simulink model "conversion"  (Simulink 10.1)
settings: Solver=FixedStepDiscrete  StartTime=0.0  StopTime=10.0  FixedStep=0.1  RelTol=1e-3  EnableMultiTasking=on
settings Model: Creator=Demos  LastModifiedBy=MaximeBe
settings DataIOCC: LimitDataPoints=on  SignalLoggingSaveFormat=ModelDataLogs
settings OptimizationCC: ExpressionDepthLimit=2147483647  ZeroExternalMemoryAtStartup=off  ZeroInternalMemoryAtStartup=off  LifeSpan=auto
settings DebuggingCC: SolverPrmCheckMsg=warning  FcnCallInpInsideContextMsg=warning  StateNameClashWarn=warning  SFExecutionAtInitializationDiag=warning
settings HardwareCC: ProdBitPerPointer=64  ProdBitPerSizeT=64  ProdBitPerPtrDiffT=64  ProdLargestAtomicFloat=Float  ProdIntDivRoundTo=Zero  ProdEndianess=LittleEndian  ProdWordSize=64  ProdHWDeviceType=Intel->x86-64 (Windows64)  TargetBitPerPointer=64  TargetBitPerSizeT=64  TargetBitPerPtrDiffT=64  TargetLongLongMode=on  TargetIntDivRoundTo=Zero  TargetEndianess=LittleEndian  TargetWordSize=64  TargetHWDeviceType=MATLAB Host  ProdEqTarget=off
settings RTWCC: Description=Generate an RTMaps component embedding the model  SystemTargetFile=rtmaps.tlc  TemplateMakefile=rtmaps_default_tmf  PostCodeGenCommand=rtmaps_post_code_generation(buildInfo)  RetainRTWFile=on  TargetLang=C++
settings STFCustomTargetCC: ModelReferenceCompliant=off  ConcurrentExecutionCompliant=on  CombineOutputUpdateFcns=on  MultiInstanceERTCode=on  CodeInterfacePackaging=C++ class  CPPClassGenCompliant=on  GRTInterface=off  SystemTargetFile=rtmaps.tlc
settings GRTTargetCC: ModelReferenceCompliant=off  ParMdlRefBuildCompliant=off  CompOptLevelCompliant=off  CombineOutputUpdateFcns=on  MatFileLogging=off  MultiInstanceERTCode=on  CodeInterfacePackaging=C++ class  GRTInterface=off  UseToolchainInfoCompliant=off
settings CPPComponent: GenerateDestructor=on  ExternalIOMemberVisibility=private  GenerateExternalIOAccessMethods=Inlined structure-based method  ParameterMemberVisibility=public  InternalMemberVisibility=private  GenerateParameterAccessMethods=None  GenerateInternalMemberAccessMethods=None  UseOperatorNewForModelRefRegistration=off  IncludeModelTypesInModelClass=on

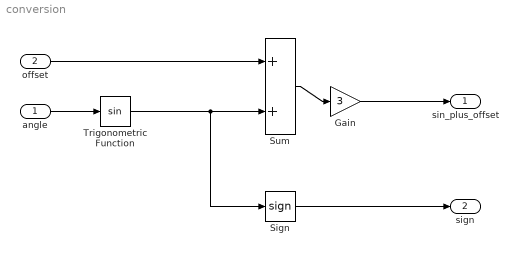
== system conversion ==
  angle : Inport
  offset : Inport  Port=2
  Gain : Gain  Gain=3
  Sign : Signum
  Sum : Sum
  Trigonometric Function : Trigonometry
  sin_plus_offset : Outport
  sign : Outport  Port=2
  wires:
  angle/1 -> Trigonometric Function/1
  Gain/1 -> sin_plus_offset/1
  Sign/1 -> sign/1
  Sum/1 -> Gain/1
  offset/1 -> Sum/1
  Trigonometric Function/1 -> Sum/2, Sign/1
